simulink library "landinggear_lib"  (Simulink 6.6)
libraries: simulink x2
settings Model: Creator=amurch  LastModifiedBy=cox  ExtModeAutoUpdateStatusClock=off

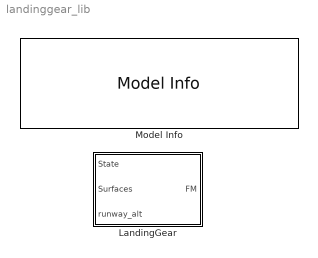
== system landinggear_lib ==
  LandingGear : Subsystem  mask(LandingGear){GEAR_SPRING=25*12, zeta=0.4, NoseWheelRate=0.15}
      mask prompts: GEAR_SPRING "Gear Spring Constant (lbs/ft)"; zeta "Damping Factor"; NoseWheelRate "Nose Wheel Sensitivity"
      mask help: Landing Gear Model
  Model Info : simulink/Model-Wide Utilities/Model Info  SystemSampleTime=-1  InitialBlockCM=None  BlockCM=None  Frame=on  DisplayStringWithTags=|  HorizontalTextAlignment=Center  LeftAlignmentValue=0.5  SourceBlockDiagram=landinggear_lib  TagMaxNumber=20
      | Landing Gear Library
      | %<ModelVersion>
      | Las modified by %<LastModifiedBy> on %<LastModificationDate>

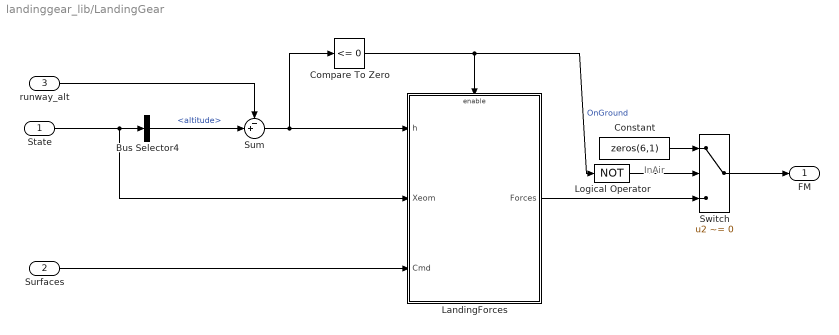
== system landinggear_lib/LandingGear ==
  note: InAir
  State : Inport
  Surfaces : Inport  Port=2
  runway_alt : Inport  Port=3
  Bus Selector4 : BusSelector  OutputSignals=altitude
  Compare To Zero : simulink/Logic and Bit Operations/Compare To Zero  SystemSampleTime=-1  relop=<=  LogicOutDataTypeMode=boolean  ZeroCross=off
  Constant : Constant  Value=zeros(6,1)
  LandingForces : Subsystem
  Logical Operator : Logic  Operator=NOT  AllPortsSameDT=off  OutDataTypeMode=Boolean
  Sum : Sum  Inputs=-+|
  Switch : Switch  Criteria=u2 ~= 0  Threshold=.5
  FM : Outport
  wires:
  Logical Operator/1 -> Switch/2
  Constant/1 -> Switch/1
  LandingForces/1(Forces) -> Switch/3
  Switch/1 -> FM/1
  Compare To Zero/1 -> Logical Operator/1, LandingForces/Enable  "OnGround"
  Surfaces/1 -> LandingForces/3(Cmd)
  Sum/1 -> LandingForces/1(h), Compare To Zero/1
  Bus Selector4/1 -> Sum/2  "<altitude>"
  State/1 -> LandingForces/2(Xeom), Bus Selector4/1
  runway_alt/1 -> Sum/1

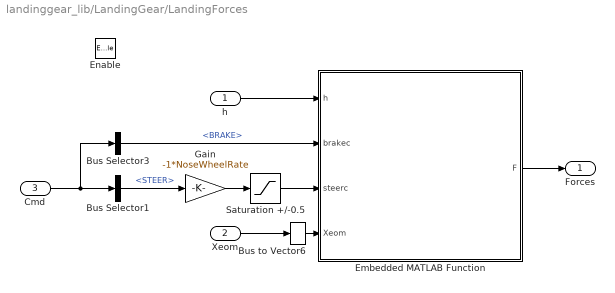
== system landinggear_lib/LandingGear/LandingForces ==
  h : Inport
  Xeom : Inport  Port=2
  Cmd : Inport  Port=3
  Enable : EnablePort
  Bus Selector1 : BusSelector  OutputSignals=STEER
  Bus Selector3 : BusSelector  OutputSignals=BRAKE
  Bus to Vector6 : BusToVector
  Embedded MATLAB Function : Stateflow chart
  Gain : Gain  Gain=-1*NoseWheelRate
  Saturation +/-0.5 : Saturate
  Forces : Outport  InitialOutput=zeros(6,1)
  wires:
  Bus Selector3/1 -> Embedded MATLAB Function/2(brakec)  "<BRAKE>"
  Bus Selector1/1 -> Gain/1  "<STEER>"
  Cmd/1 -> Bus Selector1/1, Bus Selector3/1
  Embedded MATLAB Function/1(F) -> Forces/1
  Xeom/1 -> Bus to Vector6/1
  h/1 -> Embedded MATLAB Function/1(h)
  Gain/1 -> Saturation +/-0.5/1
  Saturation +/-0.5/1 -> Embedded MATLAB Function/3(steerc)
  Bus to Vector6/1 -> Embedded MATLAB Function/4(Xeom)

== matlab function LandingGear/LandingForces/Embedded MATLAB Function ==
  data: h input inherited; brakec input inherited; steerc input inherited; Xeom input inherited; F output inherited; GEAR_SPRING parameter inherited; zeta parameter inherited
function F = fcn(h,brakec,steerc,Xeom,GEAR_SPRING,zeta)
% This block supports an embeddable subset of the MATLAB language.
% See the help menu for details. 

BRAKE_DAMPER=5;  %lbf sec/ft
MAX_BRAKES=20;   %lbf

K=GEAR_SPRING*[1;2;1] ;  % lbs*ft/rad; roll, pitch, yaw (Landing Gear Geometry)
GEAR_DAMPER=2*zeta*sqrt(GEAR_SPRING*50); %assume 50 lbs aircraft
C=2*zeta*sqrt(K*50);  %  assume 50 lbs aircraft

uvw=Xeom(1:3);
pqr=Xeom(4:6);
euler=Xeom(10:12);

% Brakes act as damper, with saturation in x, always on in y
% Z force is spring on relative height, damper on vertical velocity
% Torques are spring/damper on euler angles, with psi relative to steering reference
F=[ -1*sign(uvw(1))*max(brakec*BRAKE_DAMPER*abs(uvw(1)),BRAKE_DAMPER);...
    -1*sign(uvw(2))*max(BRAKE_DAMPER*abs(uvw(2)),BRAKE_DAMPER);...
     GEAR_SPRING*h - GEAR_DAMPER*uvw(3);
    -K.*(euler(:)-[0;0;euler(3)]) - C.*pqr(:) + K/2.*[0;0;steerc] ];
